simulink model "ThermalControl"  (R2025a)
settings: Solver=FixedStepDiscrete  StartTime=0.0  StopTime=10000  FixedStep=0.1  RelTol=1e-3
undefined symbols (not defined in the file): CtrlThrBattTrgTemp, CtrlThrEMTrgTemp
libraries: simulink x1
settings Model: DataDictionary=VirtualVehicleTemplate.sldd  ModifiedByFormat=The MathWorks, Inc.  Creator=The MathWorks, Inc.  LastModifiedBy=The MathWorks, Inc.
settings SolverCC: PositivePriorityOrder=on  AutoInsertRateTranBlk=on
settings RTWCC: GPUComputeCapability=3.5

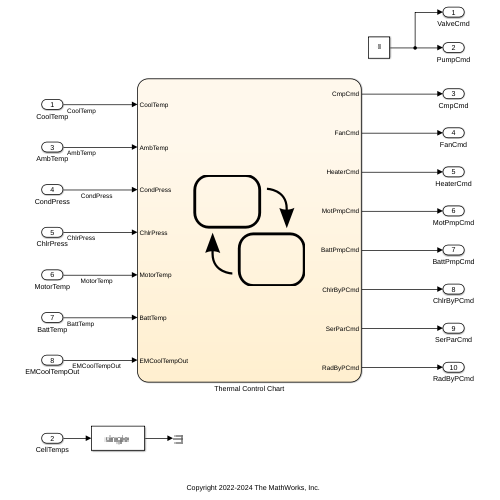
[thumbnail: Simulink's stored preview of the top-level diagram]
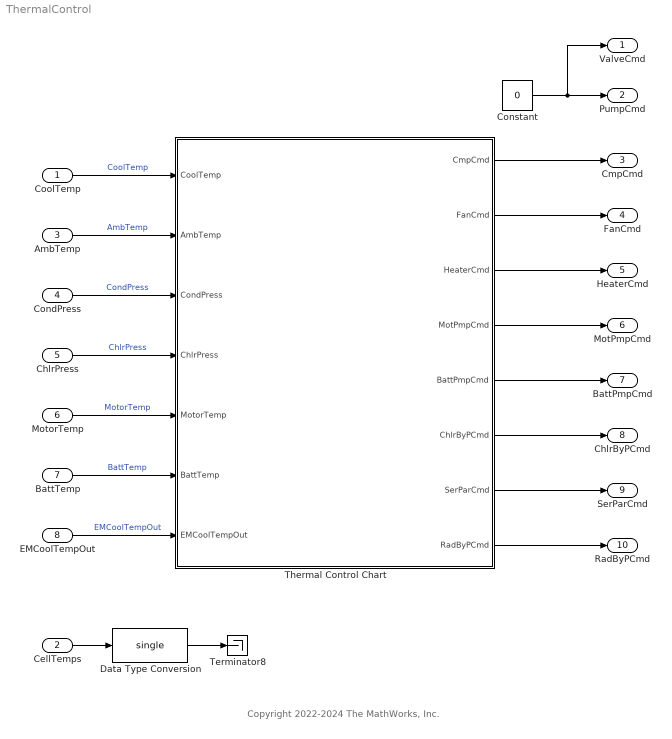
== system ThermalControl ==
  note: Copyright 2022-2024 The MathWorks, Inc.
  CoolTemp : Inport  Unit=K
  CellTemps : Inport  Port=2  PortDimensions=PlntBattNumCellSer
  AmbTemp : Inport  Port=3  Unit=K
  CondPress : Inport  Port=4  Unit=MPa
  ChlrPress : Inport  Port=5  Unit=MPa
  MotorTemp : Inport  Port=6  Unit=K
  BattTemp : Inport  Port=7  Unit=K
  EMCoolTempOut : Inport  Port=8  Unit=K
  Constant : Constant  Value=0  SampleTime=0.1
  Data Type Conversion : DataTypeConversion  OutDataTypeStr=single  SaturateOnIntegerOverflow=off  RndMeth=Floor
  Terminator8 : Terminator
  Thermal Control Chart : Stateflow chart  TreatAsAtomicUnit=on
      settings: PortSchema="{\"entries\":[{\"content\":{\"sides\":[{\"content\":{\"connectorIds\":[\"In3\",\"In1\",\"In7\",\"In6\",\"In5\",\"In2\",\"In4\"]},\"type\":\"ConnectorPlacement.EquallySpacedRectSide\",\"uuid\":\"4fe00f39-37c1-46c0-a616-5b099423e3d7\"},{\"content\":{\"connectorIds\":[\"Out7\",\"Out8\",\"Out6\",\"Out5\",\"Out1\",\"Out2\",\"Out4\",\"Out3\"],\"side\":\"RIGHT\"},\"type\":\"ConnectorPlacement.EquallySpacedRectSide\",\"uuid\":\"6ae0ae8a-110b-42ac-9a90-d19ce2f3e627\"},{\"content\":{\"side\":\"TOP\"},\"type\":\"ConnectorPlacement.EquallySpacedRectSide\",\"uuid\":\"967ec737-ce44-4288-a966-e7dea48843da\"}]},\"type\":\"ConnectorPlacement.EquallySpacedConnector\",\"uuid\":\"2306cd3b-afc9-459a-bc9d-49ac1ff51bed\"}],\"packageUris\":[\"http://schema.mathworks.com/mf0/Connector/R2020b\"],\"version\":\"1.0\"}"
  ValveCmd : Outport
  PumpCmd : Outport  Port=2
  CmpCmd : Outport  Port=3
  FanCmd : Outport  Port=4
  HeaterCmd : Outport  Port=5
  MotPmpCmd : Outport  Port=6
  BattPmpCmd : Outport  Port=7
  ChlrByPCmd : Outport  Port=8
  SerParCmd : Outport  Port=9
  RadByPCmd : Outport  Port=10
  wires:
  AmbTemp/1 -> Thermal Control Chart/1(AmbTemp)  "AmbTemp"
  CondPress/1 -> Thermal Control Chart/7(CondPress)  "CondPress"
  BattTemp/1 -> Thermal Control Chart/2(BattTemp)  "BattTemp"
  EMCoolTempOut/1 -> Thermal Control Chart/4(EMCoolTempOut)  "EMCoolTempOut"
  CoolTemp/1 -> Thermal Control Chart/3(CoolTemp)  "CoolTemp"
  MotorTemp/1 -> Thermal Control Chart/5(MotorTemp)  "MotorTemp"
  Thermal Control Chart/1(BattPmpCmd) -> BattPmpCmd/1
  Thermal Control Chart/2(ChlrByPCmd) -> ChlrByPCmd/1
  Thermal Control Chart/5(MotPmpCmd) -> MotPmpCmd/1
  Thermal Control Chart/4(SerParCmd) -> SerParCmd/1
  Thermal Control Chart/3(RadByPCmd) -> RadByPCmd/1
  Thermal Control Chart/6(HeaterCmd) -> HeaterCmd/1
  Thermal Control Chart/7(CmpCmd) -> CmpCmd/1
  ChlrPress/1 -> Thermal Control Chart/6(ChlrPress)  "ChlrPress"
  Thermal Control Chart/8(FanCmd) -> FanCmd/1
  Constant/1 -> ValveCmd/1, PumpCmd/1
  Data Type Conversion/1 -> Terminator8/1
  CellTemps/1 -> Data Type Conversion/1

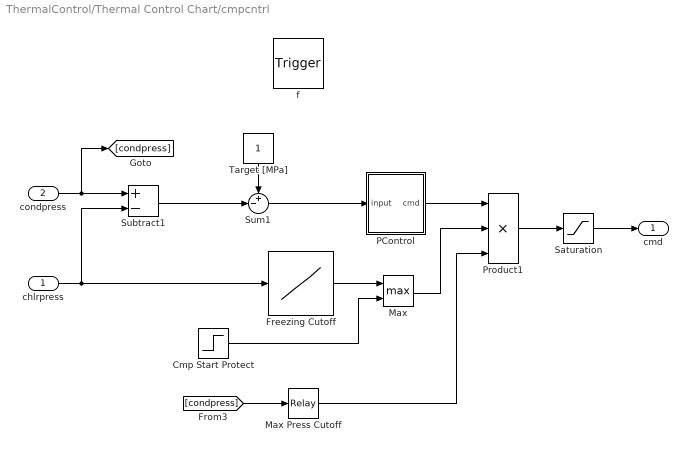
== system ThermalControl/Thermal Control Chart/cmpcntrl ==
  chlrpress : Inport  OutDataTypeStr=double  PortDimensions=1
  condpress : Inport  Port=2  OutDataTypeStr=double  PortDimensions=1
  f : TriggerPort  TriggerType=function-call  VariantControl=(inherit)  SampleTime=-1
      settings: CopyFcn=Stateflow.SLINSF.SimulinkMan.removeBlockPreDeleteFcn  PreDeleteFcn=Stateflow.SLINSF.SimulinkMan.unsafePredeleteFcn
  Cmp Start Protect : Step  Time=15  Before=1  After=0
  Freezing Cutoff : Lookup_n-D  NumberOfTableDimensions=1  BreakpointsForDimension1=[0.3 0.31]  IndexSearchMethod=Linear search  BeginIndexSearchUsingPreviousIndexResult=on  Table=[0.1 1]  ExtrapMethod=Clip  InternalRulePriority=Speed  RndMeth=Simplest
  Max : MinMax  Function=max  Inputs=2
  Max Press Cutoff : Relay  OnSwitchValue=3  OffSwitchValue=2.9  OnOutputValue=0.1  OffOutputValue=1
  PControl : Subsystem
  Product1 : Product  Inputs=3
  Saturation : Saturate  UpperLimit=1  LowerLimit=0.1
  Subtract1 : Sum  Inputs=+-
  Sum1 : Sum  Inputs=+-|
  Target [MPa] : Constant
  cmd : Outport
  wires:
  Target [MPa]/1 -> Sum1/1
  Cmp Start Protect/1 -> Max/2
  Max/1 -> Product1/2
  Saturation/1 -> cmd/1
  PControl/1(cmd) -> Product1/1
  [condpress] -> Max Press Cutoff/1
  Max Press Cutoff/1 -> Product1/3
  Freezing Cutoff/1 -> Max/1
  Sum1/1 -> PControl/1(input)
  Product1/1 -> Saturation/1
  Subtract1/1 -> Sum1/2
  condpress/1 -> [condpress], Subtract1/1
  chlrpress/1 -> Subtract1/2, Freezing Cutoff/1

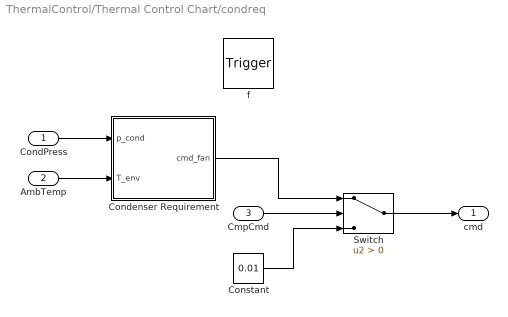
== system ThermalControl/Thermal Control Chart/condreq ==
  CondPress : Inport  OutDataTypeStr=double  PortDimensions=1
  AmbTemp : Inport  Port=2  OutDataTypeStr=double  PortDimensions=1
  CmpCmd : Inport  Port=3  OutDataTypeStr=double  PortDimensions=1
  f : TriggerPort  TriggerType=function-call  VariantControl=(inherit)  SampleTime=-1
      settings: CopyFcn=Stateflow.SLINSF.SimulinkMan.removeBlockPreDeleteFcn  PreDeleteFcn=Stateflow.SLINSF.SimulinkMan.unsafePredeleteFcn
  Condenser Requirement : Subsystem
  Constant : Constant  Value=0.01  SampleTime=-1
  Switch : Switch  Criteria=u2 > Threshold  SaturateOnIntegerOverflow=off  InputSameDT=off
  cmd : Outport
  wires:
  Switch/1 -> cmd/1
  Constant/1 -> Switch/3
  CmpCmd/1 -> Switch/2
  Condenser Requirement/1(cmd_fan) -> Switch/1
  CondPress/1 -> Condenser Requirement/1(p_cond)
  AmbTemp/1 -> Condenser Requirement/2(T_env)

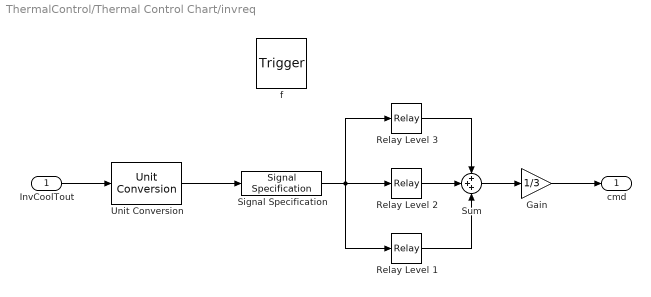
== system ThermalControl/Thermal Control Chart/invreq ==
  InvCoolTout : Inport  OutDataTypeStr=double  Unit=K  PortDimensions=1
  f : TriggerPort  TriggerType=function-call  VariantControl=(inherit)  SampleTime=-1
      settings: CopyFcn=Stateflow.SLINSF.SimulinkMan.removeBlockPreDeleteFcn  PreDeleteFcn=Stateflow.SLINSF.SimulinkMan.unsafePredeleteFcn
  Gain : Gain  Gain=1/3
  Relay Level 1 : Relay  OnSwitchValue=75  OffSwitchValue=65
  Relay Level 2 : Relay  OnSwitchValue=85  OffSwitchValue=76
  Relay Level 3 : Relay  OnSwitchValue=95  OffSwitchValue=86
  Signal Specification : SignalSpecification  Unit=°C
  Sum : Sum  Inputs=+++
  Unit Conversion : UnitConversion
  cmd : Outport
  wires:
  Relay Level 2/1 -> Sum/2
  Sum/1 -> Gain/1
  Signal Specification/1 -> Relay Level 2/1, Relay Level 3/1, Relay Level 1/1
  Relay Level 1/1 -> Sum/3
  Relay Level 3/1 -> Sum/1
  Unit Conversion/1 -> Signal Specification/1
  Gain/1 -> cmd/1
  InvCoolTout/1 -> Unit Conversion/1

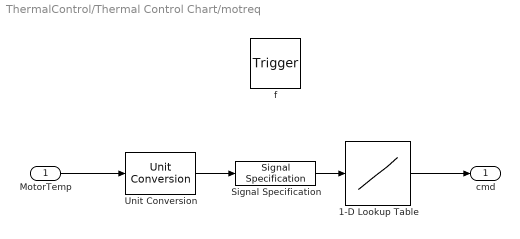
== system ThermalControl/Thermal Control Chart/motreq ==
  MotorTemp : Inport  OutDataTypeStr=double  Unit=K  PortDimensions=1
  f : TriggerPort  TriggerType=function-call  VariantControl=(inherit)  SampleTime=-1
      settings: CopyFcn=Stateflow.SLINSF.SimulinkMan.removeBlockPreDeleteFcn  PreDeleteFcn=Stateflow.SLINSF.SimulinkMan.unsafePredeleteFcn
  1-D Lookup Table : Lookup_n-D  NumberOfTableDimensions=1  BreakpointsForDimension1=[-50 45 48 52 58 60 75 130]  IndexSearchMethod=Linear search  BeginIndexSearchUsingPreviousIndexResult=on  Table=[0 0 0.1 0.3 0.5 0.7 1 1]  InternalRulePriority=Speed  RndMeth=Simplest
  Signal Specification : SignalSpecification  Unit=°C
  Unit Conversion : UnitConversion
  cmd : Outport
  wires:
  Unit Conversion/1 -> Signal Specification/1
  Signal Specification/1 -> 1-D Lookup Table/1
  1-D Lookup Table/1 -> cmd/1
  MotorTemp/1 -> Unit Conversion/1

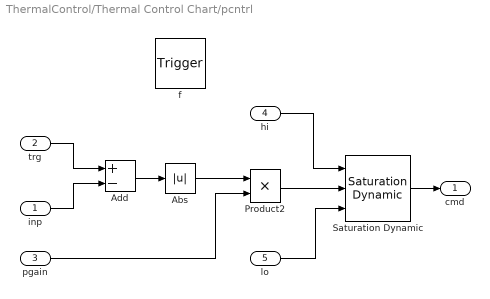
== system ThermalControl/Thermal Control Chart/pcntrl ==
  inp : Inport  OutDataTypeStr=double  PortDimensions=1
  trg : Inport  Port=2  OutDataTypeStr=double  PortDimensions=1
  pgain : Inport  Port=3  OutDataTypeStr=double  PortDimensions=1
  hi : Inport  Port=4  OutDataTypeStr=double  PortDimensions=1
  lo : Inport  Port=5  OutDataTypeStr=double  PortDimensions=1
  f : TriggerPort  TriggerType=function-call  VariantControl=(inherit)  SampleTime=-1
      settings: CopyFcn=Stateflow.SLINSF.SimulinkMan.removeBlockPreDeleteFcn  PreDeleteFcn=Stateflow.SLINSF.SimulinkMan.unsafePredeleteFcn
  Abs : Abs  SaturateOnIntegerOverflow=off
  Add : Sum  Inputs=+-
  Product2 : Product
  Saturation Dynamic : simulink/Discontinuities/Saturation Dynamic  OutMin=[]  OutMax=[]  OutDataTypeStr=Inherit: Same as second input  OutDataType=fixdt(1, 16)  OutScaling=2^-10  DoSatur=off
  cmd : Outport
  wires:
  trg/1 -> Add/1
  inp/1 -> Add/2
  Add/1 -> Abs/1
  Saturation Dynamic/1 -> cmd/1
  pgain/1 -> Product2/2
  Product2/1 -> Saturation Dynamic/2
  Abs/1 -> Product2/1
  hi/1 -> Saturation Dynamic/1
  lo/1 -> Saturation Dynamic/3

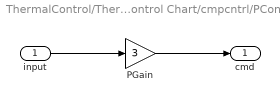
== system ThermalControl/Thermal Control Chart/cmpcntrl/PControl ==
  input : Inport
  PGain : Gain  Gain=3
  cmd : Outport
  wires:
  input/1 -> PGain/1
  PGain/1 -> cmd/1

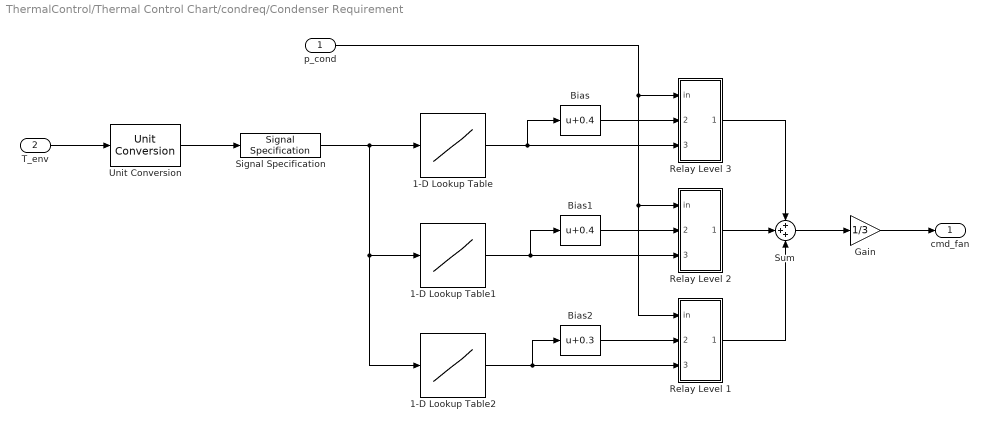
== system ThermalControl/Thermal Control Chart/condreq/Condenser Requirement ==
  p_cond : Inport
  T_env : Inport  Port=2  Unit=K
  1-D Lookup Table : Lookup_n-D  NumberOfTableDimensions=1  BreakpointsForDimension1=[0 20 30 40 50]  IndexSearchMethod=Linear search  BeginIndexSearchUsingPreviousIndexResult=on  Table=[2.0 2.0 1.8 1.5 1.3]  InternalRulePriority=Speed  RndMeth=Simplest
  1-D Lookup Table1 : Lookup_n-D  NumberOfTableDimensions=1  BreakpointsForDimension1=[0 20 30 40 50]  IndexSearchMethod=Linear search  BeginIndexSearchUsingPreviousIndexResult=on  Table=[1.4 1.4 1.3 1.2 1.1]  InternalRulePriority=Speed  RndMeth=Simplest
  1-D Lookup Table2 : Lookup_n-D  NumberOfTableDimensions=1  BreakpointsForDimension1=[0 20 30 40 50]  IndexSearchMethod=Linear search  BeginIndexSearchUsingPreviousIndexResult=on  Table=[0.8 0.8 0.8 0.8 0.8]  InternalRulePriority=Speed  RndMeth=Simplest
  Bias : Bias  Bias=0.4  SaturateOnIntegerOverflow=off
  Bias1 : Bias  Bias=0.4  SaturateOnIntegerOverflow=off
  Bias2 : Bias  Bias=0.3  SaturateOnIntegerOverflow=off
  Gain : Gain  Gain=1/3
  Relay Level 1 : Subsystem
  Relay Level 2 : Subsystem
  Relay Level 3 : Subsystem
  Signal Specification : SignalSpecification  Unit=°C
  Sum : Sum  Inputs=+++
  Unit Conversion : UnitConversion
  cmd_fan : Outport
  wires:
  Unit Conversion/1 -> Signal Specification/1
  Signal Specification/1 -> 1-D Lookup Table2/1, 1-D Lookup Table1/1, 1-D Lookup Table/1
  Gain/1 -> cmd_fan/1
  T_env/1 -> Unit Conversion/1
  Bias2/1 -> Relay Level 1/2(high)
  1-D Lookup Table2/1 -> Bias2/1, Relay Level 1/3(low)
  Bias1/1 -> Relay Level 2/2(high)
  1-D Lookup Table1/1 -> Bias1/1, Relay Level 2/3(low)
  Bias/1 -> Relay Level 3/2(high)
  1-D Lookup Table/1 -> Bias/1, Relay Level 3/3(low)
  Relay Level 1/1(out) -> Sum/3
  Relay Level 2/1(out) -> Sum/2
  Relay Level 3/1(out) -> Sum/1
  p_cond/1 -> Relay Level 1/1(in), Relay Level 2/1(in), Relay Level 3/1(in)
  Sum/1 -> Gain/1

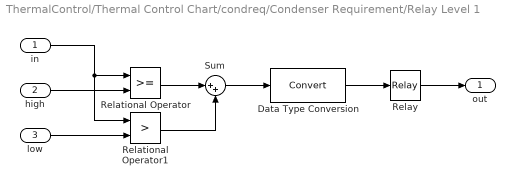
== system ThermalControl/Thermal Control Chart/condreq/Condenser Requirement/Relay Level 1 ==
  in : Inport
  high : Inport  Port=2
  low : Inport  Port=3
  Data Type Conversion : DataTypeConversion  SaturateOnIntegerOverflow=off  RndMeth=Floor
  Relational Operator : RelationalOperator  OutDataTypeStr=boolean  RndMeth=Simplest  InputSameDT=off
  Relational Operator1 : RelationalOperator  Operator=>  OutDataTypeStr=boolean  RndMeth=Simplest  InputSameDT=off
  Relay : Relay  OnSwitchValue=1.5  OffSwitchValue=0.5
  Sum : Sum  Inputs=|++
  out : Outport
  wires:
  in/1 -> Relational Operator1/1, Relational Operator/1
  high/1 -> Relational Operator/2
  low/1 -> Relational Operator1/2
  Relay/1 -> out/1
  Relational Operator/1 -> Sum/1
  Relational Operator1/1 -> Sum/2
  Data Type Conversion/1 -> Relay/1
  Sum/1 -> Data Type Conversion/1

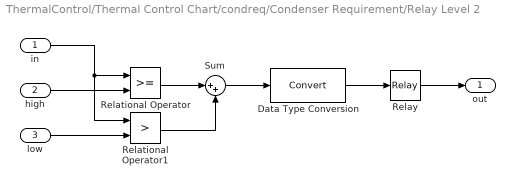
== system ThermalControl/Thermal Control Chart/condreq/Condenser Requirement/Relay Level 2 ==
  in : Inport
  high : Inport  Port=2
  low : Inport  Port=3
  Data Type Conversion : DataTypeConversion  SaturateOnIntegerOverflow=off  RndMeth=Floor
  Relational Operator : RelationalOperator  OutDataTypeStr=boolean  RndMeth=Simplest  InputSameDT=off
  Relational Operator1 : RelationalOperator  Operator=>  OutDataTypeStr=boolean  RndMeth=Simplest  InputSameDT=off
  Relay : Relay  OnSwitchValue=1.5  OffSwitchValue=0.5
  Sum : Sum  Inputs=|++
  out : Outport
  wires:
  in/1 -> Relational Operator1/1, Relational Operator/1
  high/1 -> Relational Operator/2
  low/1 -> Relational Operator1/2
  Relay/1 -> out/1
  Relational Operator/1 -> Sum/1
  Relational Operator1/1 -> Sum/2
  Data Type Conversion/1 -> Relay/1
  Sum/1 -> Data Type Conversion/1

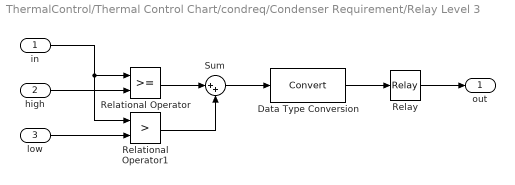
== system ThermalControl/Thermal Control Chart/condreq/Condenser Requirement/Relay Level 3 ==
  in : Inport
  high : Inport  Port=2
  low : Inport  Port=3
  Data Type Conversion : DataTypeConversion  SaturateOnIntegerOverflow=off  RndMeth=Floor
  Relational Operator : RelationalOperator  OutDataTypeStr=boolean  RndMeth=Simplest  InputSameDT=off
  Relational Operator1 : RelationalOperator  Operator=>  OutDataTypeStr=boolean  RndMeth=Simplest  InputSameDT=off
  Relay : Relay  OnSwitchValue=1.5  OffSwitchValue=0.5
  Sum : Sum  Inputs=|++
  out : Outport
  wires:
  in/1 -> Relational Operator1/1, Relational Operator/1
  high/1 -> Relational Operator/2
  low/1 -> Relational Operator1/2
  Relay/1 -> out/1
  Relational Operator/1 -> Sum/1
  Relational Operator1/1 -> Sum/2
  Data Type Conversion/1 -> Relay/1
  Sum/1 -> Data Type Conversion/1

== stateflow chart ThermalControl/Thermal Control Chart ==
  state Pumps [parallel]
    settings: executionOrder=1
    state PumpsON
      during:
      BattPmpCmd = ...
      pcntrl(BattTemp,CtrlThrBattTrgTemp,1,1,0.1);
    state PumpsOFF
      entry:
      BattPmpCmd = 0.01;
    (default) -> PumpsOFF
    PumpsOFF -> PumpsON : [BattTemp - CtrlThrBattTrgTemp > 0 || MotorTemp - CtrlThrEMTrgTemp > 3 || ...
        |  CtrlThrBattTrgTemp - AmbTemp > 20]
    PumpsON -> PumpsOFF : [CtrlThrBattTrgTemp - BattTemp > 5 && CtrlThrEMTrgTemp - MotorTemp > 5]
  state Heater [parallel]
    settings: executionOrder=2
    state HeatON
      entry:
      HeaterCmd = 1;
    state HeatOFF
      entry:
      HeaterCmd = 0;
    (default) -> HeatOFF
    HeatOFF -> HeatON : [BattPmpCmd > 0 && CtrlThrBattTrgTemp - CoolTemp > 20 && ...
        | CtrlThrBattTrgTemp - AmbTemp > 20 ]
    HeatON -> HeatOFF : [CtrlThrBattTrgTemp - CoolTemp < 10]
  state cmd = pcntrl(inp,trg,pgain,hi,lo) [function]
  state cmd = cmpcntrl(chlrpress, ... [function]
    condpress)
  state ChillerBypass [parallel]
    settings: executionOrder=3
    state ChillerON
      entry:
      ChlrByPCmd = 0;
      during:
      CmpCmd = ...
      cmpcntrl(ChlrPress,CondPress);
    state ChillerOFF
      entry:
      ChlrByPCmd = 1;
      CmpCmd = 0;
    (default) -> ChillerOFF
    ChillerOFF -> ChillerON : [HeaterCmd == 0 && BattPmpCmd > 0.01 && ...
        |  BattTemp - CtrlThrBattTrgTemp > 0 && ...
        | BattTemp - CoolTemp < 5]
    ChillerON -> ChillerOFF : [CtrlThrBattTrgTemp - BattTemp > 5 ]
  state cmd = condreq(CondPress, ... [function]
    AmbTemp,CmpCmd)
  state cmd = invreq(InvCoolTout) [function]
  state RadiatorBypass [parallel]
    settings: executionOrder=4
    state RadiatorON
      entry:
      RadByPCmd = 0;
      during:
      fcmd1 = condreq(CondPress,AmbTemp,CmpCmd);
      fcmd2 = invreq(EMCoolTempOut);
      fcmd3 = motreq(MotorTemp);
      FanCmd = max([fcmd1,fcmd2,fcmd3]);
    state RadiatorOFF
      entry:
      RadByPCmd = 1;
      during:
      FanCmd = condreq(CondPress,AmbTemp,CmpCmd);
    (default) -> RadiatorOFF
    RadiatorOFF -> RadiatorON : [HeaterCmd == 0 && BattPmpCmd > 0 && ...
        | EMCoolTempOut - CtrlThrEMTrgTemp > 0 && ...
        | EMCoolTempOut - AmbTemp > 0]
    RadiatorON -> RadiatorOFF : [AmbTemp - EMCoolTempOut > 0]
  state cmd = motreq(MotorTemp) [function]
  state SeriesParallel [parallel]
    settings: executionOrder=5
    state Parallel
      entry:
      SerParCmd = 0;
      during:
      MotPmpCmd = ...
      pcntrl(MotorTemp,CtrlThrEMTrgTemp,1,1,0.1);
    state Series
      entry:
      SerParCmd = 1;
      during:
      MotPmpCmd = BattPmpCmd;
    (default) -> Series
    Series -> Parallel : [BattPmpCmd > 0.01 && (ChlrByPCmd < 0.5 || ...
        | max(AmbTemp,EMCoolTempOut) - CtrlThrBattTrgTemp > 10 ...
        | || MotorTemp - BattTemp > 50)]
    Parallel -> Series : [max(AmbTemp,EMCoolTempOut) - CtrlThrBattTrgTemp < 5]
  data: inp function_input double size=1; trg function_input double size=1; pgain function_input double size=1; hi function_input double size=1; lo function_input double size=1; cmd function_output; chlrpress function_input double size=1; condpress function_input double size=1; cmd function_output; CondPress function_input double size=1; AmbTemp function_input double size=1; CmpCmd function_input double size=1; cmd function_output; InvCoolTout function_input double size=1; cmd function_output; MotorTemp function_input double size=1; cmd function_output; AmbTemp input double size=1; BattTemp input; CoolTemp input; EMCoolTempOut input; MotorTemp input double size=1; BattPmpCmd output; ChlrByPCmd output; RadByPCmd output; SerParCmd output; MotPmpCmd output; HeaterCmd output; CtrlThrBattTrgTemp parameter; CtrlThrEMTrgTemp parameter; CmpCmd output double size=1; ChlrPress input; CondPress input double size=1; FanCmd output double size=1; fcmd1 local; fcmd2 local; fcmd3 local
